simulink model "prac_sim"  (R2023a)
settings: Solver=VariableStepAuto  StartTime=0.0  StopTime=10.0  RelTol=1e-3
settings Model: Creator=ASUS  LastModifiedBy=ASUS

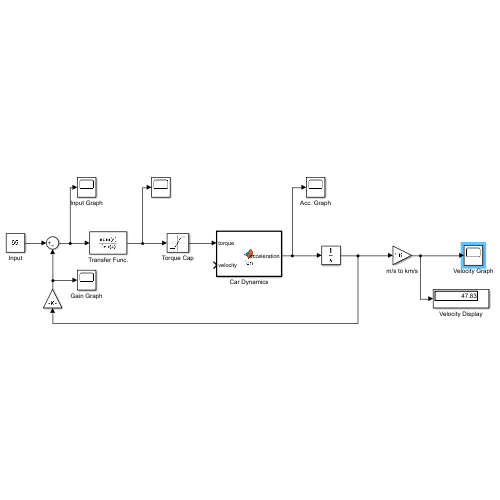
[thumbnail: Simulink's stored preview of the top-level diagram]
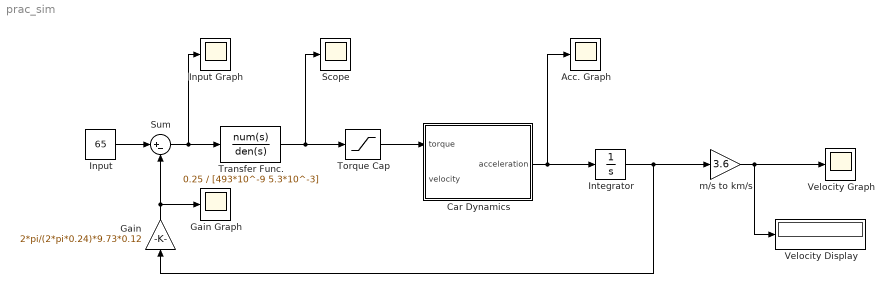
== system prac_sim ==
  Acc. Graph : Scope
  Car Dynamics : MATLAB Function  TreatAsAtomicUnit=on
  Gain : Gain  Gain=2*pi/(2*pi*0.24)*9.73*0.12
  Gain Graph : Scope
  Input : Constant  Value=65
  Input Graph : Scope
  Integrator : Integrator
  Scope : Scope
  Sum : Sum  Inputs=|+-
  Torque Cap : Saturate  UpperLimit=600  LowerLimit=0
  Transfer Func. : TransferFcn  Numerator=0.25  Denominator=[493*10^-9 5.3*10^-3]
  Velocity Display : Display
  Velocity Graph : Scope
  m/s to km/s : Gain  Gain=3.6
  wires:
  Transfer Func./1 -> Scope/1, Torque Cap/1
  Torque Cap/1 -> Car Dynamics/1(torque)
  Car Dynamics/1(acceleration) -> Integrator/1, Acc. Graph/1
  Integrator/1 -> Gain/1, m/s to km/s/1
  m/s to km/s/1 -> Velocity Display/1, Velocity Graph/1
  Sum/1 -> Input Graph/1, Transfer Func./1
  Gain/1 -> Gain Graph/1, Sum/2
  Input/1 -> Sum/1

== matlab function prac_sim/Car Dynamics ==
  data: torque input; acceleration output; velocity input
function acceleration = fcn(torque, velocity)

acceleration = (0.6 * 40.5 * torque - 413 - 0.3318 * velocity^2) / 2108;
